simulink model "mdl_example_7_5"  (R2024b)
settings: Solver=FixedStepAuto  StartTime=0.0  StopTime=T_sim  FixedStep=1  RelTol=1e-3
values from neighbouring files (symbols this model uses):
  inc = coe_sat(4)    [example_7_5_init.m]
  J5 = [6400  -76.4    -25.6 ... (first row only)    [example_7_5_init.m]
  j_min = 4726.01952    [example_7_5_init.m]
  q0 = (sqrt(2)/2)*[1 0 0 1]'    [example_7_5_init.m]
  T_orbit = 2*pi*(a_orbit^1.5)/sqrt(mu)    [example_7_5_init.m]
  w0 = [0.01 0.01 0.01]'    [example_7_5_init.m]
libraries: sharedtransform x1, simulink_extras x1
settings Model: SimulationMode=accelerator  Creator=Monster  LastModifiedBy=Monster

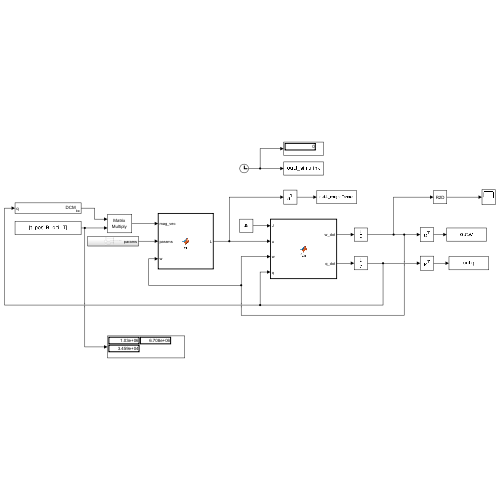
[thumbnail: Simulink's stored preview of the top-level diagram]
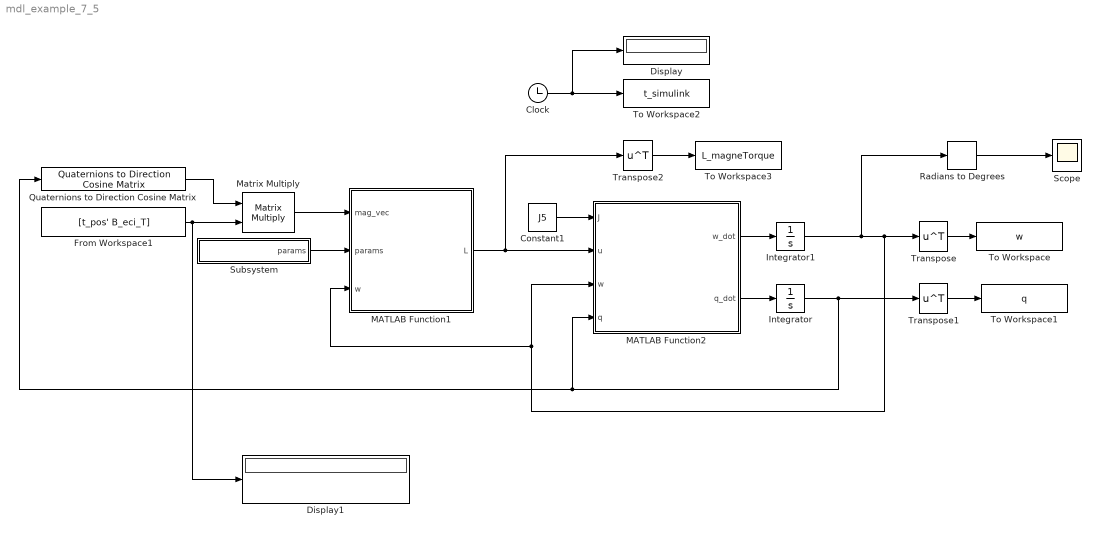
== system mdl_example_7_5 ==
  Clock : Clock
  Constant1 : Constant  Value=J5
  Display : Display
  Display1 : Display
  From Workspace1 : FromWorkspace  VariableName=[t_pos' B_eci_T]  SampleTime=1
  Integrator : Integrator  InitialCondition=q0
  Integrator1 : Integrator  InitialCondition=w0
  MATLAB Function1 : MATLAB Function  TreatAsAtomicUnit=on
  MATLAB Function2 : MATLAB Function  TreatAsAtomicUnit=on
  Matrix Multiply : Product  Multiplication=Matrix(*)
  Quaternions to Direction Cosine Matrix : sharedtransform/Quaternions to  Direction Cosine Matrix  aMode=aMode
      settings: LibrarySourceBlock=|
      | aerolibtransform2/Quaternions to
      | Direction Cosine Matrix
  Radians to Degrees : simulink_extras/Transformations/Radians to Degrees
  Scope : Scope
  Subsystem : Subsystem
  To Workspace : ToWorkspace  VariableName=w  SampleTime=-1
      settings: Save2DSignal=2-D array (concatenate along first dimension)
  To Workspace1 : ToWorkspace  VariableName=q  SampleTime=-1
      settings: Save2DSignal=2-D array (concatenate along first dimension)
  To Workspace2 : ToWorkspace  VariableName=t_simulink  SampleTime=-1
      settings: Save2DSignal=2-D array (concatenate along first dimension)
  To Workspace3 : ToWorkspace  VariableName=L_magneTorque  SampleTime=-1
      settings: Save2DSignal=2-D array (concatenate along first dimension)
  Transpose : Math  Operator=transpose
  Transpose1 : Math  Operator=transpose
  Transpose2 : Math  Operator=transpose
  wires:
  Subsystem/1(params) -> MATLAB Function1/2(params)
  MATLAB Function2/1(w_dot) -> Integrator1/1
  Constant1/1 -> MATLAB Function2/1(J)
  Transpose/1 -> To Workspace/1
  Integrator/1 -> Quaternions to Direction Cosine Matrix/1, MATLAB Function2/4(q), Transpose1/1
  Transpose1/1 -> To Workspace1/1
  MATLAB Function2/2(q_dot) -> Integrator/1
  MATLAB Function1/1(L) -> MATLAB Function2/2(u), Transpose2/1
  Clock/1 -> Display/1, To Workspace2/1
  Transpose2/1 -> To Workspace3/1
  From Workspace1/1 -> Matrix Multiply/2, Display1/1
  Quaternions to Direction Cosine Matrix/1 -> Matrix Multiply/1
  Matrix Multiply/1 -> MATLAB Function1/1(mag_vec)
  Integrator1/1 -> Radians to Degrees/1, Transpose/1, MATLAB Function2/3(w), MATLAB Function1/3(w)
  Radians to Degrees/1 -> Scope/1

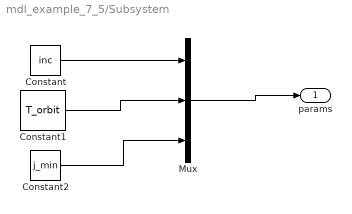
== system mdl_example_7_5/Subsystem ==
  Constant : Constant  Value=inc
  Constant1 : Constant  Value=T_orbit
  Constant2 : Constant  Value=j_min
  Mux : Mux  Inputs=3
  params : Outport
  wires:
  Constant/1 -> Mux/1
  Constant1/1 -> Mux/2
  Constant2/1 -> Mux/3
  Mux/1 -> params/1

== matlab function mdl_example_7_5/MATLAB Function1 ==
  data: mag_vec input; params input; w input; L output
function L = fcn(mag_vec, params, w)

inc = params(1);
inc = inc - deg2rad(11.5);
t_orbit = params(2);
j_min = params(3);

k = (4*pi/t_orbit)*(1+sin(inc))*j_min;

b_unit = mag_vec/norm(mag_vec);

m = -(k/norm(mag_vec))*cross(b_unit,w);

L = cross(m,mag_vec);


end

== matlab function mdl_example_7_5/MATLAB Function2 ==
  data: w_dot output; J input; u input; q_dot output; w input; q input
function [w_dot,q_dot] = fcn(J,u,w,q)


w1 = w(1);
w2 = w(2);
w3 = w(3);

W = [0,w3,-w2,w1; -w3, 0, w1, w2; w2, -w1, 0, w3; -w1, -w2, -w3, 0];
% output
w_dot = inv(J)*(u-cross(w,J*w));

q_dot = 0.5*W*q;

end
